simulink model "Fuel_Cell"  (R2023b)
settings: Solver=ode1  StartTime=0.0  StopTime=100  FixedStep=0.02  RelTol=1e-3  AbsTol=1e-3  EnableMultiTasking=on
model workspace: external: MATLAB File model_workspace.m (data not in the file)
values from neighbouring files (symbols this model uses):
  anode_tube_D = 0.004    [model_workspace.m]
  cathode_tube_D = 0.004    [model_workspace.m]
  env_p = 0.101325    [model_workspace.m]
  env_T = 60    [model_workspace.m]
  Ki_valve = 0.0005    [model_workspace.m]
  Kp_valve = 5E-5    (= 5e-05)    [model_workspace.m]
  N2_T = [-56.55 -50 -40 -30 -20 -10 -5 -4 -3 -2 -1 0 1 2 3 4 5 10 20 30          40 50 60 70 80 90 100 110 120 130 140 150 160 170 180 190 200 210          220 230 240 250 260 270 280 290 300 310 320 330 340 350]    [model_workspace.m]
  radiator_air_area_fins = 11.5625    [model_workspace.m]
  radiator_air_area_primary = 1.2231250000000002    (= 1.223125)    [model_workspace.m]
  radiator_eta_fin = 0.7    [model_workspace.m]
  radiator_rho = 2700    [model_workspace.m]
  radiator_t_wall = 0.0001    [model_workspace.m]
  stack_area = 49    [model_workspace.m]
  stack_iL = 1.4    [model_workspace.m]
  stack_mea_rho = 1800    [model_workspace.m]
  stack_num_cells = 8    [model_workspace.m]
  stack_num_channels = 1    [model_workspace.m]
  stack_t_gdl = 250    [model_workspace.m]
  stack_t_membrane = 125    [model_workspace.m]
  stack_w_channels = 0.4    [model_workspace.m]
  time_step = 0.02    [model_workspace.m]
libraries: fl_lib x108, nesl_utility x48, simulink x10
(part 1 of 3)
settings Model: Creator=The MathWorks, Inc.  LastModifiedBy=danie
settings ConfigSet: Description=VeriStand Targets (Windows & NI Linux Real-Time 64-bit)
settings SolverCC: AutoScaleAbsTol=off  MaxConsecutiveMinStep=2  AlgebraicLoopSolver=TrustRegion  AutoInsertRateTranBlk=on  InsertRTBMode=Always  MaxZcPerStep=1
settings DataIOCC: SaveOutput=off  SaveTime=off  ReturnWorkspaceOutputs=off
settings OptimizationCC: DefaultParameterBehavior=Inlined  EnhancedBackFolding=on  PassReuseOutputArgsAs=Individual arguments  ZeroExternalMemoryAtStartup=off  ZeroInternalMemoryAtStartup=off  OptimizeBlockOrder=speed  DifferentSizesBufferReuse=on  OptimizationCustomize=off  EfficientTunableParamExpr=on
settings DebuggingCC: ParameterTunabilityLossMsg=error  UnconnectedInputMsg=warning  UnconnectedOutputMsg=warning  UnconnectedLineMsg=warning  SymbolicDimsDataTypeCodeGenerationDiagnostic=none
settings HardwareCC: ProdBitPerLong=64  ProdHWDeviceType=Intel->x86-64 (Linux 64)
settings ModelReferenceCC: EnableRefExpFcnMdlSchedulingChecks=on
settings SFSimCC: MATLABDynamicMemAlloc=off  CustomCodeUndefinedFunction=UseInterfaceOnly
settings RTWCC: Description=Embedded Coder  SystemTargetFile=ert.tlc  GenCodeOnly=on  PackageGeneratedCodeAndArtifacts=on  TemplateMakefile=ert_default_tmf  BuildConfiguration=Faster Runs  DLArmComputeVersion=19.05
settings CodeAppCC: ForceParamTrailComments=on  IgnoreCustomStorageClasses=off  OperatorAnnotations=on  SimulinkDataObjDesc=on  SFDataObjDesc=on  InsertBlockDesc=on
settings ERTTargetCC: TargetLangStandard=C99 (ISO)  GenerateSampleERTMain=on  SupportContinuousTime=on  InlinedParameterPlacement=NonHierarchical  ERTCustomFileTemplate=example_file_process.tlc
settings SimscapeCC: SimscapeLogName=simlog_ssc_fuel_cell  SimscapeLogDataHistory=20000

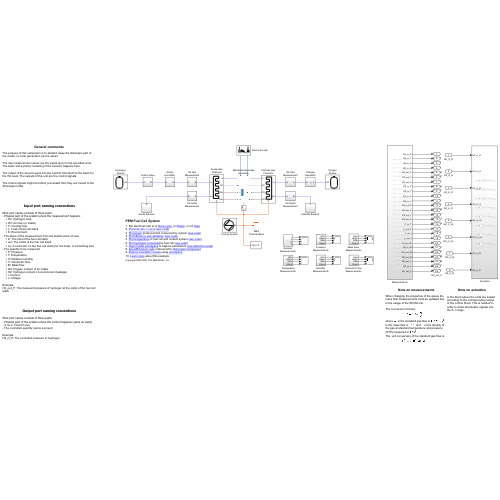
[thumbnail: Simulink's stored preview of the top-level diagram]
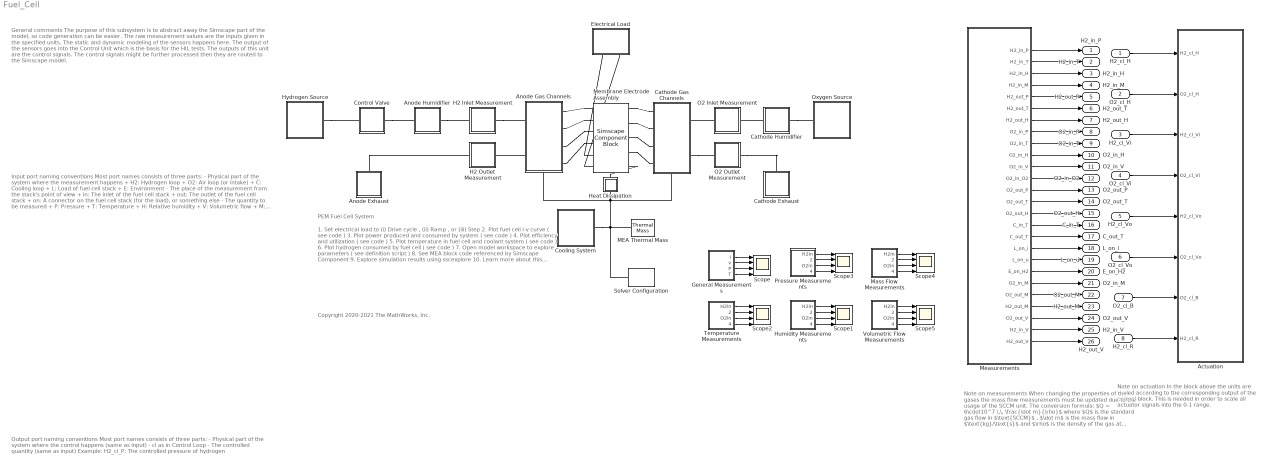
== system Fuel_Cell ==
  note: Note on actuation
      |
      | In the block above the units are scaled according to the corresponding output of the control block. This is needed in order to scale all actuator signals into the 0-1 range.
  note: Note on measurements
      |
      | When changing the properties of the gases the mass flow measurements must be updated due to the usage of the SCCM unit.
      |
      | The conversion formula:
      | $Q = 6\cdot10^7 \,\, \frac{\dot m}{\rho}$
      | where $Q$ is the standard gas flow in $\text{SCCM}$ , $\dot m$ is the mass flow in $\text{kg}/\text{s}$ and $\rho$ is the density of the gas at standard temperature and pressure (STP) measured in ${\text{kg}}/{\text{m}^3}$ .
      | The unit conversion of the standard gas flow is
      | $1 \frac{\text{m}^3}{\text{s}} = 6\cdot10^7 \,\,\text{SCCM}$
  note: PEM Fuel Cell System
  note: 1. Set electrical load to (i) Drive cycle , (ii) Ramp , or (iii) Step
      | 2. Plot fuel cell i-v curve ( see code )
      | 3. Plot power produced and consumed by system ( see code )
      | 4. Plot efficiency and utilization ( see code )
      | 5. Plot temperature in fuel cell and coolant system ( see code )
      | 6. Plot hydrogen consumed by fuel cell ( see code )
      | 7. Open model workspace to explore parameters ( see definition script )
      | 8. See MEA block code referenced by Simscape Component
      | 9. Explore simulation results using sscexplore
      | 10. Learn more about this example
  note: Copyright 2020-2021 The MathWorks, Inc.
  note: General comments
      |
      | The purpose of this subsystem is to abstract away the Simscape part of the model, so code generation can be easier.
      |
      | The raw measurement values are the inputs given in the specified units. The static and dynamic modeling of the sensors happens here.
      |
      | The output of the sensors goes into the Control Unit which is the basis for the HIL tests. The outputs of this unit are the control signals.
      |
      | The control signals might be further processed then they are routed to the Simscape model.
  note: Input port naming conventions
      |
      | Most port names consists of three parts:
      | - Physical part of the system where the measurement happens
      | + H2: Hydrogen loop
      | + O2: Air loop (or intake)
      | + C: Cooling loop
      | + L: Load of fuel cell stack
      | + E: Environment
      | - The place of the measurement from the stack's point of view
      | + in: The inlet of the fuel cell stack
      | + out: The outlet of the fuel cell stack
      | + on: A connector on the fuel cell stack (for the load), or something else
      | - The quantity to be measured
      | + P: Pressure
      | + T: Temperature
      | + H: Relative humidity
      | + V: Volumetric flow
      | + M: Mass flow
      | + O2: Oxygen content of air intake
      | + H2: Hydrogen content of environment (leakage)
      | + i: Current
      | + u: Voltage
      |
      | Example:
      | H2_out_P: The measuerd pressure of hydrogen at the outlet of the fuel cell stack
  note: Output port naming conventions
      |
      | Most port names consists of three parts:
      | - Physical part of the system where the control happens (same as input)
      | - cl as in Control Loop
      | - The controlled quantity (same as input)
      |
      | Example:
      | H2_cl_P: The controlled pressure of hydrogen
  H2_cl_H : Inport  OutDataTypeStr=double  PortDimensions=[1 1]  SampleTime=[time_step,0]
  O2_cl_H : Inport  Port=2  OutDataTypeStr=double  PortDimensions=[1 1]  SampleTime=[time_step,0]
  H2_cl_Vi : Inport  Port=3  OutDataTypeStr=double  PortDimensions=1  SampleTime=[time_step,0]
  O2_cl_Vi : Inport  Port=4  OutDataTypeStr=double  PortDimensions=1  SampleTime=[time_step,0]
  H2_cl_Vo : Inport  Port=5  OutDataTypeStr=double  PortDimensions=1  SampleTime=[time_step,0]
  O2_cl_Vo : Inport  Port=6  OutDataTypeStr=double  PortDimensions=1  SampleTime=[time_step,0]
  O2_cl_B : Inport  Port=7  OutDataTypeStr=double  PortDimensions=1  SampleTime=[time_step,0]
  H2_cl_R : Inport  Port=8  OutDataTypeStr=double  PortDimensions=1  SampleTime=[time_step,0]
  Actuation : Subsystem
  Anode Humidifier : Subsystem  Tag=PublishSubsystem
  Anode Exhaust : Subsystem  Tag=PublishSubsystem
      settings: PortSchema="{\"entries\":[{\"content\":{\"sides\":[{\"content\":{\"connectorIds\":[]},\"type\":\"ConnectorPlacement.EquallySpacedRectSide\",\"uuid\":\"6344d1cf-22ea-4a51-9588-07afca0fac15\"},{\"content\":{\"connectorIds\":[],\"side\":\"RIGHT\"},\"type\":\"ConnectorPlacement.EquallySpacedRectSide\",\"uuid\":\"a3908f81-9410-4056-87cd-9faba76d3fb8\"},{\"content\":{\"connectorIds\":[\"LConn1\"],\"side\":\"TOP\"},\"type\":\"ConnectorPlacement.EquallySpacedRectSide\",\"uuid\":\"a1c9e24d-adb9-4361-8e9b-feafccbbdb81\"}]},\"type\":\"ConnectorPlacement.EquallySpacedConnector\",\"uuid\":\"d5180d8f-18a0-491d-9fff-909db43c9aea\"}],\"packageUris\":[\"http://schema.mathworks.com/mf0/Connector/R2020b\"],\"version\":\"1.0\"}"
  Anode Gas Channels : Subsystem  Tag=PublishSubsystem
      settings: PortSchema="{\"entries\":[{\"content\":{\"sides\":[{\"content\":{\"connectorIds\":[\"LConn1\",\"LConn2\"]},\"type\":\"ConnectorPlacement.EquallySpacedRectSide\",\"uuid\":\"f0c92738-2de1-40ac-9e4a-670524600aa2\"},{\"content\":{\"connectorIds\":[\"RConn1\",\"RConn2\",\"RConn3\",\"RConn4\"],\"side\":\"RIGHT\"},\"type\":\"ConnectorPlacement.EquallySpacedRectSide\",\"uuid\":\"f0ed995d-2dce-4bd6-9faa-b1cb502a30b1\"},{\"content\":{\"connectorIds\":[],\"side\":\"TOP\"},\"type\":\"ConnectorPlacement.EquallySpacedRectSide\",\"uuid\":\"b5d2d698-46b6-42b5-a767-bb9f1790aa28\"},{\"content\":{\"connectorIds\":[\"RConn5\"],\"side\":\"BOTTOM\"},\"type\":\"ConnectorPlacement.EquallySpacedRectSide\",\"uuid\":\"3e8c99a3-0044-43a9-bacb-b652445e4ac6\"}]},\"type\":\"ConnectorPlacement.EquallySpacedConnector\",\"uuid\":\"912925fb-ca80-4fe6-8a1d-a2308cfd6f88\"}],\"packageUris\":[\"http://schema.mathworks.com/mf0/Connector/R2020b\"],\"version\":\"1.0\"}"
      mask Display:
      | plot(0, 0)
      | plot(100, 100)
      | 
      | x1 = 25;
      | x2 = 65;
      | y1 = 23;
      | y2 = 95;
      | xt = 15;
      | yt = 9;
      | 
      | x_pattern = [x2 x2    x1+xt x1+xt   x1+xt   x2     ];
      | y_pattern = [y2 y2-yt y2-yt y2-2*yt y2-2*yt y2-2*yt];
      | 
      | plot([x1 x1 x2 x_pattern x_pattern      x_pattern      x_pattern         x2    x1], ...
      |      [y1-yt y2 y2 y_pattern y_pattern-2*yt y_pattern-4*yt y_pattern-6*yt y1-yt y1-yt])
  Cathode Humidifier : Subsystem  Tag=PublishSubsystem
  Cathode Exhaust : Subsystem  Tag=PublishSubsystem
      settings: PortSchema="{\"entries\":[{\"content\":{\"sides\":[{\"content\":{\"connectorIds\":[]},\"type\":\"ConnectorPlacement.EquallySpacedRectSide\",\"uuid\":\"6344d1cf-22ea-4a51-9588-07afca0fac15\"},{\"content\":{\"connectorIds\":[],\"side\":\"RIGHT\"},\"type\":\"ConnectorPlacement.EquallySpacedRectSide\",\"uuid\":\"a3908f81-9410-4056-87cd-9faba76d3fb8\"},{\"content\":{\"connectorIds\":[\"LConn1\"],\"side\":\"TOP\"},\"type\":\"ConnectorPlacement.EquallySpacedRectSide\",\"uuid\":\"a1c9e24d-adb9-4361-8e9b-feafccbbdb81\"}]},\"type\":\"ConnectorPlacement.EquallySpacedConnector\",\"uuid\":\"d5180d8f-18a0-491d-9fff-909db43c9aea\"}],\"packageUris\":[\"http://schema.mathworks.com/mf0/Connector/R2020b\"],\"version\":\"1.0\"}"
  Cathode Gas Channels : Subsystem  Tag=PublishSubsystem
      settings: PortSchema="{\"entries\":[{\"content\":{\"sides\":[{\"content\":{\"connectorIds\":[\"LConn1\",\"LConn2\",\"LConn3\",\"LConn4\"]},\"type\":\"ConnectorPlacement.EquallySpacedRectSide\",\"uuid\":\"d09155df-6760-40de-80f3-d532399b6b43\"},{\"content\":{\"connectorIds\":[\"RConn1\",\"RConn2\"],\"side\":\"RIGHT\"},\"type\":\"ConnectorPlacement.EquallySpacedRectSide\",\"uuid\":\"8f76bd4e-30c2-4c8b-860a-78c10353bd22\"},{\"content\":{\"connectorIds\":[],\"side\":\"TOP\"},\"type\":\"ConnectorPlacement.EquallySpacedRectSide\",\"uuid\":\"7de91a32-4f26-479e-bbec-b6009a288b8f\"},{\"content\":{\"connectorIds\":[\"RConn3\"],\"side\":\"BOTTOM\"},\"type\":\"ConnectorPlacement.EquallySpacedRectSide\",\"uuid\":\"b696b46e-4734-4c8a-bae1-7c8793078c6b\"}]},\"type\":\"ConnectorPlacement.EquallySpacedConnector\",\"uuid\":\"30d7c265-b676-4649-8112-8a94c6c095da\"}],\"packageUris\":[\"http://schema.mathworks.com/mf0/Connector/R2020b\"],\"version\":\"1.0\"}"
      mask Display:
      | plot(0, 0)
      | plot(100, 100)
      | 
      | x1 = 35;
      | x2 = 75;
      | y1 = 23;
      | y2 = 95;
      | xt = 15;
      | yt = 9;
      | 
      | x_pattern = [x1 x1    x2-xt x2-xt   x2-xt   x1     ];
      | y_pattern = [y2 y2-yt y2-yt y2-2*yt y2-2*yt y2-2*yt];
      | 
      | plot([x2 x2 x1 x_pattern x_pattern      x_pattern      x_pattern         x1    x2], ...
      |      [y1-yt y2 y2 y_pattern y_pattern-2*yt y_pattern-4*yt y_pattern-6*yt y1-yt y1-yt])
  Control Valve : Subsystem  Tag=PublishSubsystem
  Cooling System : Subsystem  Tag=PublishSubsystem
      mask Display:
      | plot(0, 0)
      | plot(100, 100)
      | 
      | n = 80;
      | r = 35;
      | 
      | x = 45;
      | y = 50;
      | t = 5;
      | 
      | plot(cos(linspace(0, 2*pi, n))*r + x, sin(linspace(0, 2*pi, n))*r + y)
      | 
      | plot([x x x-r+t x+r-t x x], [y+r+2*t y+r-t y y y-r+t y-r-2*t])
  Electrical Load : Subsystem  Tag=PublishSubsystem  mask(Electrical Load){input_type=Drive cycle}
      mask prompts: input_type "Select one of the following scenarios:"
      settings: PortSchema="{\"entries\":[{\"content\":{\"sides\":[{\"content\":{\"connectorIds\":[]},\"type\":\"ConnectorPlacement.EquallySpacedRectSide\",\"uuid\":\"cf26c57a-4aaa-4eca-a1cf-dab3379228b7\"},{\"content\":{\"connectorIds\":[],\"side\":\"RIGHT\"},\"type\":\"ConnectorPlacement.EquallySpacedRectSide\",\"uuid\":\"bd4a28c6-f8d3-4492-9f61-a12eb17ccdd3\"},{\"content\":{\"connectorIds\":[],\"side\":\"TOP\"},\"type\":\"ConnectorPlacement.EquallySpacedRectSide\",\"uuid\":\"7f54a4db-ccf4-4e3a-a135-4ada067d241f\"},{\"content\":{\"connectorIds\":[\"RConn1\",\"RConn2\"],\"side\":\"BOTTOM\"},\"type\":\"ConnectorPlacement.EquallySpacedRectSide\",\"uuid\":\"8817983d-3f79-43b3-9594-6d12f7dcf066\"}]},\"type\":\"ConnectorPlacement.EquallySpacedConnector\",\"uuid\":\"79253ea6-cd7f-4983-840a-f5cee3a4dd91\"}],\"packageUris\":[\"http://schema.mathworks.com/mf0/Connector/R2020b\"],\"version\":\"1.0\"}"
      mask TypeOptions input_type: Drive cycle | Current Ramp | Current Step | Current Ramped Step | Power Ramped Step
      mask Callback input_type:
      | activeVariant = get_param(gcb, 'input_type');
      | set_param([gcb '/Inputs'], 'OverrideUsingVariant', activeVariant)
      mask Display:
      | blk = get_param([gcb, '/Inputs'], 'CompiledActiveChoiceBlock');
      | eval(get_param(blk, 'MaskDisplay'))
  General Measurements : Subsystem
  H2 Inlet Measurement : Subsystem  Tag=PublishSubsystem
  H2 Outlet Measurement : Subsystem  Tag=PublishSubsystem
  Heat Dissipation : Subsystem
      settings: PortSchema="{\"entries\":[{\"content\":{\"sides\":[{\"content\":{\"connectorIds\":[]},\"type\":\"ConnectorPlacement.EquallySpacedRectSide\",\"uuid\":\"40b2385a-b20e-464f-8016-3228e4acac4a\"},{\"content\":{\"connectorIds\":[],\"side\":\"RIGHT\"},\"type\":\"ConnectorPlacement.EquallySpacedRectSide\",\"uuid\":\"0e95dc4b-d2da-4ab6-a6e9-e2cb275776ce\"},{\"content\":{\"connectorIds\":[\"LConn1\"],\"side\":\"TOP\"},\"type\":\"ConnectorPlacement.EquallySpacedRectSide\",\"uuid\":\"0f5995c7-26f6-433d-889b-dea78bcd2b2a\"},{\"content\":{\"connectorIds\":[\"RConn1\"],\"side\":\"BOTTOM\"},\"type\":\"ConnectorPlacement.EquallySpacedRectSide\",\"uuid\":\"a2ee1c19-f9e9-4dbd-a9ff-92feea387e85\"}]},\"type\":\"ConnectorPlacement.EquallySpacedConnector\",\"uuid\":\"721753ea-9ada-4c74-8c6f-50b905d96904\"}],\"packageUris\":[\"http://schema.mathworks.com/mf0/Connector/R2020b\"],\"version\":\"1.0\"}"
  Humidity Measurements : Subsystem
  Hydrogen Source : Subsystem  Tag=PublishSubsystem
      mask Display:
      | plot(0, 0)
      | plot(100, 100)
      | 
      | n = 20;
      | r = 20;
      | x1 = 15;
      | x2 = 65;
      | y1 = 5;
      | y2 = 85;
      | 
      | plot([x1 x1], [y1+r y2-r])
      | plot([x1+r x2-r], [y2 y2])
      | plot([x2 x2], [y2-r y1+r])
      | plot([x2-r x1+r], [y1 y1])
      | 
      | plot(cos(linspace(pi/2, pi, n))*r + x1+r, sin(linspace(pi/2, pi, n))*r + y2-r)
      | plot(cos(linspace(0, pi/2, n))*r + x2-r, sin(linspace(0, pi/2, n))*r + y2-r)
      | plot(cos(linspace(3*pi/2, 2*pi, n))*r + x2-r, sin(linspace(3*pi/2, 2*pi, n))*r + y1+r)
      | plot(cos(linspace(pi, 3*pi/2, n))*r + x1+r, sin(linspace(pi, 3*pi/2, n))*r + y1+r)
      | 
      | plot([-5 -5 5 5] + (x1+x2)/2, [0 5 5 0] + y2)
  MEA Thermal Mass : fl_lib/Thermal/Thermal Elements/Thermal Mass  mass_type=foundation.enum.constant_variable.constant  mass=stack_mea_rho * stack_area*1e-4 * (stack_t_membrane + 2*stack_t_gdl)*1e-6 * stack_num_cells kg  sp_heat=stack_mea_cp J/kg/K  mass_min=1e-6 kg  num_ports=foundation.enum.numPorts2.one  m_specify=off  m_priority=High  m=1 kg  m_nominal_specify=off  m_nominal_unit=kg  m_nominal_value=1  T_specify=on  T_priority=High  T=env_T degC  T_nominal_specify=off  T_nominal_unit=K  T_nominal_value=1  Q_specify=off  Q_priority=None  Q=0 W  Q_nominal_specify=off  Q_nominal_unit=W  Q_nominal_value=1
  Mass Flow Measurements : Subsystem
  Measurements : Subsystem
  Membrane Electrode Assembly : SimscapeComponentBlock  SourceFile=FuelCell  ComponentPath=FuelCell  ComponentVariants="[\"FuelCell\"]"  ComponentVariantNames="[\"FuelCell\"]"  ClassName=FuelCell  SchemaVersion=1  N_cell=stack_num_cells  area_cell=stack_area cm^2  t_membrane=stack_t_membrane um  t_gdl_A=stack_t_gdl um  t_gdl_C=stack_t_gdl um  io=stack_io A/cm^2  iL=stack_iL A/cm^2  alpha=stack_alpha  D_H2O_gdl_A=stack_D_gdl cm^2/s  D_H2O_gdl_C=stack_D_gdl cm^2/s  rho_membrane=stack_membrane_rho kg/m^3  M_membrane=stack_membrane_MW kg/mol  i_specify=off  i_priority=None  i=0 A  i_nominal_specify=off  i_nominal_unit=A  i_nominal_value=1  Q_specify=off  Q_priority=None  Q=0 W  Q_nominal_specify=off  Q_nominal_unit=W  Q_nominal_value=1  a_H2O_acl_specify=off  a_H2O_acl_priority=None  a_H2O_acl=0.5  a_H2O_acl_nominal_specify=off  a_H2O_acl_nominal_unit=1  a_H2O_acl_nominal_value=1  a_H2O_ccl_specify=off  a_H2O_ccl_priority=None  a_H2O_ccl=0.5  a_H2O_ccl_nominal_specify=off  a_H2O_ccl_nominal_unit=1  a_H2O_ccl_nominal_value=1
      settings: CopyFcn=simscape.engine.sli.internal.componentblockcallback(gcbh,'COPY')  PreCopyFcn=simscape.engine.sli.internal.componentblockcallback(gcbh,'PRECOPY')  PreDeleteFcn=simscape.engine.sli.internal.componentblockcallback(gcbh,'PREDELETE')  InternalSimscapePortConfiguration="{\"Bottom\":[{\"id\":\"H\",\"label\":\"H\",\"type\":\"foundation.thermal.thermal\"}],\"Left\":[{\"id\":\"A\",\"label\":\"A\",\"type\":\"foundation.moist_air.moist_air\"},{\"id\":\"SA\",\"label\":\"SA\",\"type\":\"foundation.moist_air.moist_air_source\"},{\"id\":\"FAi\",\"label\":\"FAi\",\"type\":\"input\"},{\"id\":\"FAo\",\"label\":\"FAo\",\"type\":\"input\"}],\"Right\":[{\"id\":\"C\",\"label\":\"C\",\"type\":\"foundation.moist_air.moist_air\"},{\"id\":\"SC\",\"label\":\"SC\",\"type\":\"foundation.moist_air.moist_air_source\"},{\"id\":\"FCi\",\"label\":\"FCi\",\"type\":\"input\"},{\"id\":\"FCo\",\"label\":\"FCo\",\"type\":\"input\"}],\"Top\":[{\"id\":\"n\",\"label\":\"-\",\"type\":\"foundation.electrical.electrical\"},{\"id\":\"p\",\"label\":\"+\",\"type\":\"foundation.electrical.electrical\"}]}"
      mask Type: Fuel Cell
  O2 Inlet Measurement : Subsystem  Tag=PublishSubsystem
  O2 Outlet Measurement : Subsystem  Tag=PublishSubsystem
  Oxygen Source : Subsystem  Tag=PublishSubsystem
      mask Display:
      | plot(0, 0)
      | plot(100, 100)
      | 
      | n = 20;
      | r = 20;
      | x1 = 35;
      | x2 = 85;
      | y1 = 5;
      | y2 = 85;
      | 
      | plot([x1 x1], [y1+r y2-r])
      | plot([x1+r x2-r], [y2 y2])
      | plot([x2 x2], [y2-r y1+r])
      | plot([x2-r x1+r], [y1 y1])
      | 
      | plot(cos(linspace(pi/2, pi, n))*r + x1+r, sin(linspace(pi/2, pi, n))*r + y2-r)
      | plot(cos(linspace(0, pi/2, n))*r + x2-r, sin(linspace(0, pi/2, n))*r + y2-r)
      | plot(cos(linspace(3*pi/2, 2*pi, n))*r + x2-r, sin(linspace(3*pi/2, 2*pi, n))*r + y1+r)
      | plot(cos(linspace(pi, 3*pi/2, n))*r + x1+r, sin(linspace(pi, 3*pi/2, n))*r + y1+r)
      | 
      | plot([-5 -5 5 5] + (x1+x2)/2, [0 5 5 0] + y2)
  Pressure Measurements : Subsystem
  Scope{,1..5} (6 alike) : Scope  NumInputPorts=4
  Solver Configuration : nesl_utility/Solver Configuration  PhysicalDomain=network_engine_domain  SubClassName=solver  LeftPortType=input  RightPortType=generic  Tones=[]  Harmonics=[]  SimulateNoise=off  Profile=off  UseLocalSampling=off  EnableSwitchedLinearOptims=on  FrequencyDomain=off  UseCCode=off  RelTol=0.001  AbsTol=1e-06  MinStep=1e-09  ToWorkspace=off  RevertToSquareIcSolve=off  NumHomotopyIterations=100  PhasorMode=off  PhasorModeNumHarmonics=1  ConsistencySolver=NEWTON_FTOL  IndexReductionMethod=DerivativeReplacement  DoDC=on  ResidualTolerance=1e-05  ConsistencyTolSource=GLOBAL  ConsistencyAbsTol=0.001  ConsistencyRelTol=0.001  ConsistencyTolFactor=0.001  UseLocalSolver=on  LocalSolverChoice=NE_BACKWARD_EULER_ADVANCER  ResolveIndetEquations=on  FunctionEvalNumThread=1  LocalSolverSampleTime=time_step  DoFixedCost=off  MaxNonlinIter=3  MaxModeIter=2  ComputeImpulses=off  ImpulseIterations=2  LinearAlgebra=auto  LinearAlgebraNumThread=0  EquationFormulation=NE_TIME_EF  DelaysMemoryBudget=1024  AutomaticFiltering=on  FilteringTimeConstant=0.01  PartitionStorageMethod=AS_NEEDED  PartitionMemoryBudget=1024  PartitionMethod=ROBUST  MultibodyUseLocalSolver=off  MultibodyLocalSolverChoice=ODE1  MultibodyLocalSolverSampleTime=0.001
  Temperature Measurements : Subsystem
  Volumetric Flow Measurements : Subsystem
  H2_in_P : Outport  OutDataTypeStr=double  PortDimensions=[1 1]  SampleTime=[time_step,0]
  H2_in_T : Outport  Port=2  OutDataTypeStr=double  PortDimensions=[1 1]  SampleTime=[time_step,0]
  H2_in_H : Outport  Port=3  OutDataTypeStr=double  PortDimensions=[1 1]  SampleTime=[time_step,0]
  H2_in_M : Outport  Port=4  OutDataTypeStr=double  PortDimensions=[1 1]  SampleTime=[time_step,0]
  H2_out_P : Outport  Port=5  OutDataTypeStr=double  PortDimensions=[1 1]  SampleTime=[time_step,0]
  H2_out_T : Outport  Port=6  OutDataTypeStr=double  PortDimensions=[1 1]  SampleTime=[time_step,0]
  H2_out_H : Outport  Port=7  OutDataTypeStr=double  PortDimensions=[1 1]  SampleTime=[time_step,0]
  O2_in_P : Outport  Port=8  OutDataTypeStr=double  PortDimensions=[1 1]  SampleTime=[time_step,0]
  O2_in_T : Outport  Port=9  OutDataTypeStr=double  PortDimensions=[1 1]  SampleTime=[time_step,0]
  O2_in_H : Outport  Port=10  OutDataTypeStr=double  PortDimensions=[1 1]  SampleTime=[time_step,0]
  O2_in_V : Outport  Port=11  OutDataTypeStr=double  PortDimensions=[1 1]  SampleTime=[time_step,0]
  O2_in_O2 : Outport  Port=12  OutDataTypeStr=double  PortDimensions=[1 1]  SampleTime=[time_step,0]
  O2_out_P : Outport  Port=13  OutDataTypeStr=double  PortDimensions=[1 1]  SampleTime=[time_step,0]
  O2_out_T : Outport  Port=14  OutDataTypeStr=double  PortDimensions=[1 1]  SampleTime=[time_step,0]
  O2_out_H : Outport  Port=15  OutDataTypeStr=double  PortDimensions=[1 1]  SampleTime=[time_step,0]
  C_in_T : Outport  Port=16  OutDataTypeStr=double  PortDimensions=1  SampleTime=[time_step,0]
  C_out_T : Outport  Port=17  OutDataTypeStr=double  PortDimensions=1  SampleTime=[time_step,0]
  L_on_i : Outport  Port=18  OutDataTypeStr=double  PortDimensions=1  SampleTime=[time_step,0]
  L_on_u : Outport  Port=19  OutDataTypeStr=double  PortDimensions=1  SampleTime=[time_step,0]
  E_on_H2 : Outport  Port=20  OutDataTypeStr=double  PortDimensions=1  SampleTime=[time_step,0]
  O2_in_M : Outport  Port=21  OutDataTypeStr=double  PortDimensions=[1 1]  SampleTime=[time_step,0]
  O2_out_M : Outport  Port=22  OutDataTypeStr=double  PortDimensions=[1 1]  SampleTime=[time_step,0]
  H2_out_M : Outport  Port=23  OutDataTypeStr=double  PortDimensions=[1 1]  SampleTime=[time_step,0]
  O2_out_V : Outport  Port=24  OutDataTypeStr=double  PortDimensions=[1 1]  SampleTime=[time_step,0]
  H2_in_V : Outport  Port=25  OutDataTypeStr=double  PortDimensions=[1 1]  SampleTime=[time_step,0]
  H2_out_V : Outport  Port=26  OutDataTypeStr=double  PortDimensions=[1 1]  SampleTime=[time_step,0]
  wires:
  H2_cl_Vi/1 -> Actuation/3(H2_cl_Vi)
  Temperature Measurements/2(H2out) -> Scope2/2
  Pressure Measurements/1(H2in) -> Scope3/1
  General Measurements/3(P) -> Scope/3
  Measurements/7(H2_out_H) -> H2_out_H/1
  Measurements/14(O2_out_T) -> O2_out_T/1
  Temperature Measurements/3(O2in) -> Scope2/3
  Measurements/13(O2_out_P) -> O2_out_P/1
  Measurements/21(O2_in_M) -> O2_in_M/1
  Pressure Measurements/4(O2out) -> Scope3/4
  General Measurements/2(v) -> Scope/2
  Humidity Measurements/2(H2out) -> Scope1/2
  General Measurements/4(T) -> Scope/4
  Measurements/26(H2_out_V) -> H2_out_V/1
  Volumetric Flow Measurements/4(O2out) -> Scope5/4
  Measurements/10(O2_in_H) -> O2_in_H/1
  Pressure Measurements/2(H2out) -> Scope3/2
  Humidity Measurements/1(H2in) -> Scope1/1
  Volumetric Flow Measurements/1(H2in) -> Scope5/1
  O2_cl_H/1 -> Actuation/2(O2_cl_H)
  Measurements/22(O2_out_M) -> O2_out_M/1
  Mass Flow Measurements/3(O2in) -> Scope4/3
  Measurements/12(O2_in_O2) -> O2_in_O2/1
  Volumetric Flow Measurements/2(H2out) -> Scope5/2
  Measurements/3(H2_in_H) -> H2_in_H/1
  Mass Flow Measurements/2(H2out) -> Scope4/2
  Pressure Measurements/3(O2in) -> Scope3/3
  Humidity Measurements/4(O2out) -> Scope1/4
  Mass Flow Measurements/1(H2in) -> Scope4/1
  Measurements/9(O2_in_T) -> O2_in_T/1
  H2_cl_H/1 -> Actuation/1(H2_cl_H)
  Mass Flow Measurements/4(O2out) -> Scope4/4
  Volumetric Flow Measurements/3(O2in) -> Scope5/3
  Temperature Measurements/4(O2out) -> Scope2/4
  Humidity Measurements/3(O2in) -> Scope1/3
  General Measurements/1(i) -> Scope/1
  Temperature Measurements/1(H2in) -> Scope2/1
  Measurements/4(H2_in_M) -> H2_in_M/1
  Measurements/6(H2_out_T) -> H2_out_T/1
  Measurements/2(H2_in_T) -> H2_in_T/1
  Measurements/1(H2_in_P) -> H2_in_P/1
  Measurements/16(C_in_T) -> C_in_T/1
  Measurements/17(C_out_T) -> C_out_T/1
  Measurements/20(E_on_H2) -> E_on_H2/1
  Measurements/11(O2_in_V) -> O2_in_V/1
  Measurements/8(O2_in_P) -> O2_in_P/1
  Measurements/18(L_on_i) -> L_on_i/1
  Measurements/5(H2_out_P) -> H2_out_P/1
  Measurements/15(O2_out_H) -> O2_out_H/1
  Measurements/25(H2_in_V) -> H2_in_V/1
  Measurements/23(H2_out_M) -> H2_out_M/1
  Measurements/19(L_on_u) -> L_on_u/1
  Measurements/24(O2_out_V) -> O2_out_V/1
  O2_cl_Vi/1 -> Actuation/4(O2_cl_Vi)
  H2_cl_Vo/1 -> Actuation/5(H2_cl_Vo)
  O2_cl_Vo/1 -> Actuation/6(O2_cl_Vo)
  O2_cl_B/1 -> Actuation/7(O2_cl_B)
  H2_cl_R/1 -> Actuation/8(H2_cl_R)
  connections:
  MEA Thermal Mass/LConn1 -- Cooling System/RConn1 -- Cathode Gas Channels/RConn3 -- Anode Gas Channels/RConn5 -- Heat Dissipation/RConn1 -- Solver Configuration/RConn1
  Membrane Electrode Assembly/LConn6 -- Electrical Load/RConn2
  Hydrogen Source/RConn1 -- Control Valve/LConn1
  Membrane Electrode Assembly/RConn1 -- Cathode Gas Channels/LConn1
  Membrane Electrode Assembly/LConn2 -- Anode Gas Channels/RConn2
  Anode Exhaust/LConn1 -- H2 Outlet Measurement/LConn1
  Membrane Electrode Assembly/LConn3 -- Anode Gas Channels/RConn3
  Membrane Electrode Assembly/RConn2 -- Cathode Gas Channels/LConn2
  Membrane Electrode Assembly/LConn4 -- Anode Gas Channels/RConn4
  Cathode Gas Channels/RConn2 -- O2 Outlet Measurement/LConn1
  Cathode Humidifier/RConn1 -- Oxygen Source/RConn1
  Membrane Electrode Assembly/RConn5 -- Heat Dissipation/LConn1
  O2 Outlet Measurement/RConn1 -- Cathode Exhaust/LConn1
  Membrane Electrode Assembly/LConn1 -- Anode Gas Channels/RConn1
  H2 Inlet Measurement/RConn1 -- Anode Gas Channels/LConn1
  O2 Inlet Measurement/LConn1 -- Cathode Gas Channels/RConn1
  Cathode Humidifier/LConn1 -- O2 Inlet Measurement/RConn1
  Anode Gas Channels/LConn2 -- H2 Outlet Measurement/RConn1
  Membrane Electrode Assembly/RConn3 -- Cathode Gas Channels/LConn3
  Membrane Electrode Assembly/LConn5 -- Electrical Load/RConn1
  Membrane Electrode Assembly/RConn4 -- Cathode Gas Channels/LConn4
  Anode Humidifier/RConn1 -- H2 Inlet Measurement/LConn1
  Control Valve/RConn1 -- Anode Humidifier/LConn1

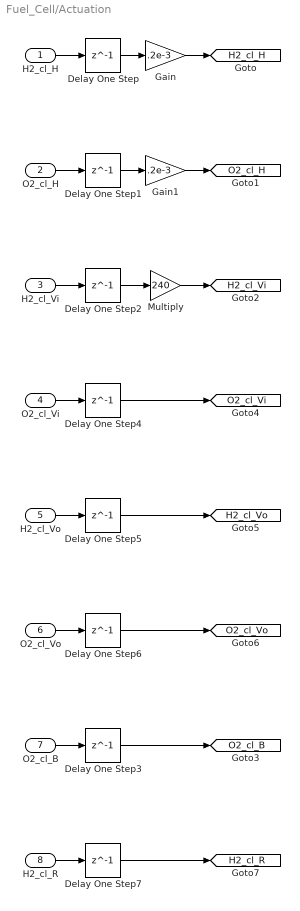
== system Fuel_Cell/Actuation ==
  H2_cl_H : Inport
  O2_cl_H : Inport  Port=2
  H2_cl_Vi : Inport  Port=3
  O2_cl_Vi : Inport  Port=4
  H2_cl_Vo : Inport  Port=5
  O2_cl_Vo : Inport  Port=6
  O2_cl_B : Inport  Port=7
  H2_cl_R : Inport  Port=8
  Delay One Step{,1..7} (8 alike) : Delay  DelayLength=1
  Gain : Gain  Gain=.2e-3
  Gain1 : Gain  Gain=.2e-3
  Multiply : Gain  Gain=240
  tag scope: H2_cl_H=global, H2_cl_R=global, H2_cl_Vi=global, H2_cl_Vo=global, O2_cl_B=global, O2_cl_H=global, O2_cl_Vi=global, O2_cl_Vo=global
  wires:
  Delay One Step4/1 -> [O2_cl_Vi]
  Delay One Step3/1 -> [O2_cl_B]
  Delay One Step2/1 -> Multiply/1
  Delay One Step1/1 -> Gain1/1
  Delay One Step/1 -> Gain/1
  O2_cl_H/1 -> Delay One Step1/1
  H2_cl_H/1 -> Delay One Step/1
  Gain/1 -> [H2_cl_H]
  Gain1/1 -> [O2_cl_H]
  O2_cl_B/1 -> Delay One Step3/1
  O2_cl_Vi/1 -> Delay One Step4/1
  H2_cl_Vi/1 -> Delay One Step2/1
  Multiply/1 -> [H2_cl_Vi]
  H2_cl_Vo/1 -> Delay One Step5/1
  Delay One Step6/1 -> [O2_cl_Vo]
  O2_cl_Vo/1 -> Delay One Step6/1
  Delay One Step5/1 -> [H2_cl_Vo]
  H2_cl_R/1 -> Delay One Step7/1
  Delay One Step7/1 -> [H2_cl_R]

== system Fuel_Cell/Anode Humidifier ==
  Constant Volume Chamber (MA) : fl_lib/Moist Air/Elements/Constant Volume Chamber (MA)  volume=1 l  num_ports=foundation.enum.num_ports.two  area_A=pi*anode_tube_D^2/4 m^2  area_B=pi*anode_tube_D^2/4 m^2  area_C=0.01 m^2  area_D=0.01 m^2  RH_ws=1  time_constant=1e-3 s  moisture_trace_gas_source=foundation.enum.moisture_trace_gas_source.controlled  moisture_source_spec=foundation.enum.moisture_source_spec.vapor  moisture_mass_flow=0 kg/s  moisture_temperature_spec=foundation.enum.temperature_spec.atmospheric  moisture_temperature=293.15 K  trace_gas_mass_flow=0 kg/s  trace_gas_temperature_spec=foundation.enum.temperature_spec.atmospheric  trace_gas_temperature=293.15 K  p_I_specify=on  p_I_priority=High  p_I=0.101325 MPa  p_I_nominal_specify=off  p_I_nominal_unit=MPa  p_I_nominal_value=1  T_I_specify=on  T_I_priority=High  T_I=env_T degC  T_I_nominal_specify=off  T_I_nominal_unit=K  T_I_nominal_value=1  RH_I_specify=off  RH_I_priority=High  RH_I=0  RH_I_nominal_specify=off  RH_I_nominal_unit=1  RH_I_nominal_value=1  x_w_I_specify=off  x_w_I_priority=None  x_w_I=0  x_w_I_nominal_specify=off  x_w_I_nominal_unit=1  x_w_I_nominal_value=1  y_w_I_specify=off  y_w_I_priority=None  y_w_I=0  y_w_I_nominal_specify=off  y_w_I_nominal_unit=1  y_w_I_nominal_value=1  HR_I_specify=off  HR_I_priority=None  HR_I=0  HR_I_nominal_specify=off  HR_I_nominal_unit=1  HR_I_nominal_value=1  x_g_I_specify=on  x_g_I_priority=None  x_g_I=0  x_g_I_nominal_specify=off  x_g_I_nominal_unit=1  x_g_I_nominal_value=1  y_g_I_specify=on  y_g_I_priority=High  y_g_I=tank_yH2  y_g_I_nominal_specify=off  y_g_I_nominal_unit=1  y_g_I_nominal_value=1
      settings: InternalSimscapePortConfiguration="{\"Bottom\":[],\"Left\":[{\"id\":\"A\",\"label\":\"A\",\"type\":\"foundation.moist_air.moist_air\"},{\"id\":\"B\",\"label\":\"B\",\"type\":\"foundation.moist_air.moist_air\"}],\"Right\":[{\"id\":\"W\",\"label\":\"W\",\"type\":\"output\"},{\"id\":\"F\",\"label\":\"F\",\"type\":\"output\"},{\"id\":\"H\",\"label\":\"H\",\"type\":\"foundation.thermal.thermal\"},{\"id\":\"S\",\"label\":\"S\",\"type\":\"foundation.moist_air.moist_air_source\"}],\"Top\":[]}"
  Controlled Moisture Source (MA) : fl_lib/Moist Air/Sources/Moisture & Trace Gas Sources/Moisture Source (MA)  source_type=foundation.enum.constant_controlled.controlled  moisture_source_spec=foundation.enum.moisture_source_spec.vapor  moisture_mass_flow=0 kg/s  temperature_spec=foundation.enum.temperature_spec.atmospheric  moisture_temperature=293.15 K  Phi_S_specify=off  Phi_S_priority=None  Phi_S=0 kW  Phi_S_nominal_specify=off  Phi_S_nominal_unit=kW  Phi_S_nominal_value=1  mdot_w_S_specify=off  mdot_w_S_priority=None  mdot_w_S=0 kg/s  mdot_w_S_nominal_specify=off  mdot_w_S_nominal_unit=kg/s  mdot_w_S_nominal_value=1
      settings: InternalSimscapePortConfiguration="{\"Bottom\":[],\"Left\":[{\"id\":\"S\",\"label\":\"S\",\"type\":\"foundation.moist_air.moist_air_source\"}],\"Right\":[{\"id\":\"M\",\"label\":\"M\",\"type\":\"input\"},{\"id\":\"T\",\"label\":\"T\",\"type\":\"input\"}],\"Top\":[]}"
  Convective Heat Transfer : fl_lib/Thermal/Thermal Elements/Convective Heat Transfer  thermal_type=foundation.enum.constant_variable.constant  area=0.5 m^2  heat_tr_coeff=900 W/(m^2 * K)  min_heat_tr_coeff=1e-3 W/(K*m^2)  T_specify=off  T_priority=None  T=0 K  T_nominal_specify=off  T_nominal_unit=K  T_nominal_value=1  Q_specify=off  Q_priority=None  Q=0 W  Q_nominal_specify=off  Q_nominal_unit=W  Q_nominal_value=1
  Delay One Step : Delay  DelayLength=1
  Environment Temperature : fl_lib/Thermal/Thermal Sources/Temperature Source  temperature=env_T degC
  Simulink-PS Converter : nesl_utility/Simulink-PS Converter  PhysicalDomain=network_engine_domain  SubClassName=ps_input  LeftPortType=input  RightPortType=output  PseudoPeriodic=off  Frequencies=[]  NoiseDistribution=none  NoiseParameters=[]  Unit=kg/s  AffineConversion=off  FilteringAndDerivatives=provide  SimscapeFilterOrder=1  InputFilterTimeConstant=0.001  UdotUserProvided=0
  Simulink-PS Converter1 : nesl_utility/Simulink-PS Converter  PhysicalDomain=network_engine_domain  SubClassName=ps_input  LeftPortType=input  RightPortType=output  PseudoPeriodic=off  Frequencies=[]  NoiseDistribution=none  NoiseParameters=[]  Unit=degC  AffineConversion=on  FilteringAndDerivatives=provide  SimscapeFilterOrder=1  InputFilterTimeConstant=0.001  UdotUserProvided=0
  A : PMIOPort  Side=Left
  B : PMIOPort  Port=2  Side=Right
  wires:
  Delay One Step/1 -> Simulink-PS Converter1/1
  [H2_cl_H] -> Simulink-PS Converter/1
  [T_stack] -> Delay One Step/1
  connections:
  Environment Temperature/LConn1 -- Convective Heat Transfer/RConn1
  Constant Volume Chamber (MA)/LConn1 -- A/RConn1
  Constant Volume Chamber (MA)/LConn2 -- B/RConn1
  Convective Heat Transfer/LConn1 -- Constant Volume Chamber (MA)/RConn3
  Constant Volume Chamber (MA)/RConn4 -- Controlled Moisture Source (MA)/LConn1
  Simulink-PS Converter1/RConn1 -- Controlled Moisture Source (MA)/RConn2
  Controlled Moisture Source (MA)/RConn1 -- Simulink-PS Converter/RConn1

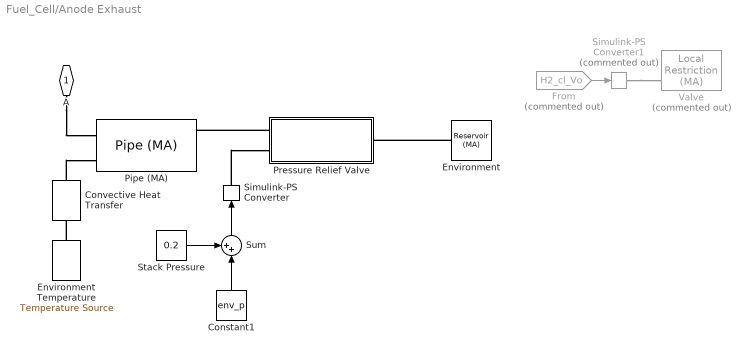
== system Fuel_Cell/Anode Exhaust ==
  Constant1 : Constant  Value=env_p
  Convective Heat Transfer : fl_lib/Thermal/Thermal Elements/Convective Heat Transfer  thermal_type=foundation.enum.constant_variable.constant  area=pi*anode_tube_D*1 m^2  heat_tr_coeff=20 W/(m^2 * K)  min_heat_tr_coeff=1e-3 W/(K*m^2)  T_specify=off  T_priority=None  T=0 K  T_nominal_specify=off  T_nominal_unit=K  T_nominal_value=1  Q_specify=off  Q_priority=None  Q=0 W  Q_nominal_specify=off  Q_nominal_unit=W  Q_nominal_value=1
  Environment : fl_lib/Moist Air/Elements/Reservoir (MA)  pressure_spec=foundation.enum.pressure_spec.specified  reservoir_pressure=env_p MPa  temperature_spec=foundation.enum.temperature_spec.specified  reservoir_temperature=env_T degC  moisture_spec=foundation.enum.moisture_spec.relative_humidity  reservoir_RH=env_RH  reservoir_x_w=0.01  reservoir_y_w=0.01  reservoir_HR=0.01  reservoir_Tw=287 K  trace_gas_spec=foundation.enum.trace_gas_spec.mole_fraction  reservoir_x_g=0.001  reservoir_y_g=env_yO2  RH_ws=1  area_A=pi*cathode_tube_D^2/4 m^2
  Environment Temperature : fl_lib/Thermal/Thermal Sources/Temperature Source  temperature=env_T degC
  From : From  Commented=on  GotoTag=H2_cl_Vo  TagVisibility=global
  Pipe (MA) : fl_lib/Moist Air/Elements/Pipe (MA)  length=1 m  area=pi*anode_tube_D^2/4 m^2  Dh=anode_tube_D m  length_add=0.1 m  roughness=15e-6 m  Re_lam=2000  Re_tur=4000  shape_factor=64  Nu_lam=3.66  wall_condensation=false  RH_ws=1  time_constant=1e-3 s  moisture_trace_gas_source=foundation.enum.moisture_trace_gas_source.none  moisture_source_spec=foundation.enum.moisture_source_spec.vapor  moisture_mass_flow=0 kg/s  moisture_temperature_spec=foundation.enum.temperature_spec.atmospheric  moisture_temperature=293.15 K  trace_gas_mass_flow=0 kg/s  trace_gas_temperature_spec=foundation.enum.temperature_spec.atmospheric  trace_gas_temperature=293.15 K  p_I_specify=on  p_I_priority=High  p_I=env_p MPa  p_I_nominal_specify=off  p_I_nominal_unit=MPa  p_I_nominal_value=1  T_I_specify=on  T_I_priority=High  T_I=env_T degC  T_I_nominal_specify=off  T_I_nominal_unit=K  T_I_nominal_value=1  RH_I_specify=off  RH_I_priority=High  RH_I=0  RH_I_nominal_specify=off  RH_I_nominal_unit=1  RH_I_nominal_value=1  x_w_I_specify=off  x_w_I_priority=None  x_w_I=0  x_w_I_nominal_specify=off  x_w_I_nominal_unit=1  x_w_I_nominal_value=1  y_w_I_specify=off  y_w_I_priority=None  y_w_I=0  y_w_I_nominal_specify=off  y_w_I_nominal_unit=1  y_w_I_nominal_value=1  HR_I_specify=off  HR_I_priority=None  HR_I=0  HR_I_nominal_specify=off  HR_I_nominal_unit=1  HR_I_nominal_value=1  x_g_I_specify=on  x_g_I_priority=None  x_g_I=0  x_g_I_nominal_specify=off  x_g_I_nominal_unit=1  x_g_I_nominal_value=1  y_g_I_specify=on  y_g_I_priority=High  y_g_I=tank_yH2  y_g_I_nominal_specify=off  y_g_I_nominal_unit=1  y_g_I_nominal_value=1
  Pressure Relief Valve : Subsystem  Tag=PublishSubsystem  mask(Pressure Relief Valve){D=anode_tube_D, r_min=1e-4, r_max=0.8, p_range=0.005}
      mask prompts: D "Connecting tube diameter (m)"; r_min "Min diameter ratio"; r_max "Max diameter ratio"; p_range "Pressure regulation range (MPa)"
      mask help: This subsystem models a pressure relief valve that maintains a set pressure at port A. The valve is normally closed. When the pressure is above the set pressure, it begins to open.
  Simulink-PS Converter : nesl_utility/Simulink-PS Converter  PhysicalDomain=network_engine_domain  SubClassName=ps_input  LeftPortType=input  RightPortType=output  PseudoPeriodic=off  Frequencies=[]  NoiseDistribution=none  NoiseParameters=[]  Unit=MPa  AffineConversion=off  FilteringAndDerivatives=provide  SimscapeFilterOrder=1  InputFilterTimeConstant=0.001  UdotUserProvided=0
  Simulink-PS Converter1 : nesl_utility/Simulink-PS Converter  Commented=on  PhysicalDomain=network_engine_domain  SubClassName=ps_input  LeftPortType=input  RightPortType=output  PseudoPeriodic=off  Frequencies=[]  NoiseDistribution=none  NoiseParameters=[]  Unit=1  AffineConversion=off  FilteringAndDerivatives=provide  SimscapeFilterOrder=1  InputFilterTimeConstant=0.001  UdotUserProvided=0
  Stack Pressure : Constant  Value=0.2
  Sum : Sum  Inputs=++|
  Valve : fl_lib/Moist Air/Elements/Local Restriction (MA)  Commented=on  restriction_type=foundation.enum.restriction_type.variable  restriction_area=0.001 m^2  min_area=pi*(1e-4*anode_tube_D)^2/4 m^2  max_area=pi*(0.8*anode_tube_D)^2/4 m^2  area=pi*anode_tube_D^2/4 m^2  Cd=0.64  B_lam=0.999
  A : PMIOPort  Side=Left
  wires:
  Stack Pressure/1 -> Sum/1
  Sum/1 -> Simulink-PS Converter/1
  Constant1/1 -> Sum/2
  From/1 -> Simulink-PS Converter1/1
  connections:
  Simulink-PS Converter/RConn1 -- Pressure Relief Valve/LConn2
  Environment Temperature/LConn1 -- Convective Heat Transfer/RConn1
  Convective Heat Transfer/LConn1 -- Pipe (MA)/LConn2
  A/RConn1 -- Pipe (MA)/LConn1
  Simulink-PS Converter1/RConn1 -- Valve/LConn2
  Pressure Relief Valve/LConn1 -- Pipe (MA)/RConn1
  Environment/LConn1 -- Pressure Relief Valve/RConn1

== system Fuel_Cell/Anode Gas Channels ==
  Pipe (MA) : fl_lib/Moist Air/Elements/Pipe (MA)  length=sqrt(stack_area) / 2 cm  area=stack_w_channels^2 * stack_num_channels * stack_num_cells cm^2  Dh=stack_w_channels cm  length_add=1 cm  roughness=15e-6 m  Re_lam=2000  Re_tur=4000  shape_factor=64  Nu_lam=3.66  wall_condensation=false  RH_ws=1  time_constant=1e-3 s  moisture_trace_gas_source=foundation.enum.moisture_trace_gas_source.none  moisture_source_spec=foundation.enum.moisture_source_spec.vapor  moisture_mass_flow=0 kg/s  moisture_temperature_spec=foundation.enum.temperature_spec.atmospheric  moisture_temperature=293.15 K  trace_gas_mass_flow=0 kg/s  trace_gas_temperature_spec=foundation.enum.temperature_spec.atmospheric  trace_gas_temperature=293.15 K  p_I_specify=on  p_I_priority=High  p_I=env_p MPa  p_I_nominal_specify=off  p_I_nominal_unit=MPa  p_I_nominal_value=1  T_I_specify=on  T_I_priority=High  T_I=env_T degC  T_I_nominal_specify=off  T_I_nominal_unit=K  T_I_nominal_value=1  RH_I_specify=off  RH_I_priority=High  RH_I=0  RH_I_nominal_specify=off  RH_I_nominal_unit=1  RH_I_nominal_value=1  x_w_I_specify=off  x_w_I_priority=None  x_w_I=0  x_w_I_nominal_specify=off  x_w_I_nominal_unit=1  x_w_I_nominal_value=1  y_w_I_specify=off  y_w_I_priority=None  y_w_I=0  y_w_I_nominal_specify=off  y_w_I_nominal_unit=1  y_w_I_nominal_value=1  HR_I_specify=off  HR_I_priority=None  HR_I=0  HR_I_nominal_specify=off  HR_I_nominal_unit=1  HR_I_nominal_value=1  x_g_I_specify=on  x_g_I_priority=None  x_g_I=0  x_g_I_nominal_specify=off  x_g_I_nominal_unit=1  x_g_I_nominal_value=1  y_g_I_specify=on  y_g_I_priority=High  y_g_I=tank_yH2  y_g_I_nominal_specify=off  y_g_I_nominal_unit=1  y_g_I_nominal_value=1
  Pipe (MA)1 : fl_lib/Moist Air/Elements/Pipe (MA)  length=sqrt(stack_area) / 2 cm  area=stack_w_channels^2 * stack_num_channels * stack_num_cells cm^2  Dh=stack_w_channels cm  length_add=1 cm  roughness=15e-6 m  Re_lam=2000  Re_tur=4000  shape_factor=64  Nu_lam=3.66  wall_condensation=false  RH_ws=1  time_constant=1e-3 s  moisture_trace_gas_source=foundation.enum.moisture_trace_gas_source.controlled  moisture_source_spec=foundation.enum.moisture_source_spec.vapor  moisture_mass_flow=0 kg/s  moisture_temperature_spec=foundation.enum.temperature_spec.atmospheric  moisture_temperature=293.15 K  trace_gas_mass_flow=0 kg/s  trace_gas_temperature_spec=foundation.enum.temperature_spec.atmospheric  trace_gas_temperature=293.15 K  p_I_specify=on  p_I_priority=High  p_I=env_p MPa  p_I_nominal_specify=off  p_I_nominal_unit=MPa  p_I_nominal_value=1  T_I_specify=on  T_I_priority=High  T_I=env_T degC  T_I_nominal_specify=off  T_I_nominal_unit=K  T_I_nominal_value=1  RH_I_specify=off  RH_I_priority=High  RH_I=0  RH_I_nominal_specify=off  RH_I_nominal_unit=1  RH_I_nominal_value=1  x_w_I_specify=off  x_w_I_priority=None  x_w_I=0  x_w_I_nominal_specify=off  x_w_I_nominal_unit=1  x_w_I_nominal_value=1  y_w_I_specify=off  y_w_I_priority=None  y_w_I=0  y_w_I_nominal_specify=off  y_w_I_nominal_unit=1  y_w_I_nominal_value=1  HR_I_specify=off  HR_I_priority=None  HR_I=0  HR_I_nominal_specify=off  HR_I_nominal_unit=1  HR_I_nominal_value=1  x_g_I_specify=on  x_g_I_priority=None  x_g_I=0  x_g_I_nominal_specify=off  x_g_I_nominal_unit=1  x_g_I_nominal_value=1  y_g_I_specify=on  y_g_I_priority=High  y_g_I=tank_yH2  y_g_I_nominal_specify=off  y_g_I_nominal_unit=1  y_g_I_nominal_value=1
      settings: InternalSimscapePortConfiguration="{\"Bottom\":[],\"Left\":[{\"id\":\"A\",\"label\":\"A\",\"type\":\"foundation.moist_air.moist_air\"},{\"id\":\"H\",\"label\":\"H\",\"type\":\"foundation.thermal.thermal\"},{\"id\":\"S\",\"label\":\"S\",\"type\":\"foundation.moist_air.moist_air_source\"}],\"Right\":[{\"id\":\"B\",\"label\":\"B\",\"type\":\"foundation.moist_air.moist_air\"},{\"id\":\"W\",\"label\":\"W\",\"type\":\"output\"},{\"id\":\"F\",\"label\":\"F\",\"type\":\"output\"}],\"Top\":[]}"
  in : PMIOPort  Side=Left
  out : PMIOPort  Port=2  Side=Left
  A : PMIOPort  Port=3  Side=Right
  SA : PMIOPort  Port=4  Side=Right
  FAi : PMIOPort  Port=5  Side=Right
  FAo : PMIOPort  Port=6  Side=Right
  H : PMIOPort  Port=7  Side=Right
  connections:
  A/RConn1 -- Pipe (MA)1/LConn1 -- Pipe (MA)/RConn1
  Pipe (MA)1/LConn3 -- SA/RConn1
  Pipe (MA)/RConn3 -- FAi/RConn1
  FAo/RConn1 -- Pipe (MA)1/RConn3
  H/RConn1 -- Pipe (MA)1/LConn2 -- Pipe (MA)/LConn2
  Pipe (MA)1/RConn1 -- out/RConn1
  Pipe (MA)/LConn1 -- in/RConn1

== system Fuel_Cell/Cathode Humidifier ==
  Constant Volume Chamber (MA) : fl_lib/Moist Air/Elements/Constant Volume Chamber (MA)  volume=1 l  num_ports=foundation.enum.num_ports.two  area_A=pi*anode_tube_D^2/4 m^2  area_B=pi*anode_tube_D^2/4 m^2  area_C=0.01 m^2  area_D=0.01 m^2  RH_ws=1  time_constant=1e-3 s  moisture_trace_gas_source=foundation.enum.moisture_trace_gas_source.controlled  moisture_source_spec=foundation.enum.moisture_source_spec.vapor  moisture_mass_flow=0 kg/s  moisture_temperature_spec=foundation.enum.temperature_spec.atmospheric  moisture_temperature=293.15 K  trace_gas_mass_flow=0 kg/s  trace_gas_temperature_spec=foundation.enum.temperature_spec.atmospheric  trace_gas_temperature=293.15 K  p_I_specify=on  p_I_priority=High  p_I=0.301325 MPa  p_I_nominal_specify=off  p_I_nominal_unit=MPa  p_I_nominal_value=1  T_I_specify=on  T_I_priority=High  T_I=env_T degC  T_I_nominal_specify=off  T_I_nominal_unit=K  T_I_nominal_value=1  RH_I_specify=off  RH_I_priority=High  RH_I=0  RH_I_nominal_specify=off  RH_I_nominal_unit=1  RH_I_nominal_value=1  x_w_I_specify=off  x_w_I_priority=None  x_w_I=0  x_w_I_nominal_specify=off  x_w_I_nominal_unit=1  x_w_I_nominal_value=1  y_w_I_specify=off  y_w_I_priority=None  y_w_I=0  y_w_I_nominal_specify=off  y_w_I_nominal_unit=1  y_w_I_nominal_value=1  HR_I_specify=off  HR_I_priority=None  HR_I=0  HR_I_nominal_specify=off  HR_I_nominal_unit=1  HR_I_nominal_value=1  x_g_I_specify=off  x_g_I_priority=None  x_g_I=0  x_g_I_nominal_specify=off  x_g_I_nominal_unit=1  x_g_I_nominal_value=1  y_g_I_specify=on  y_g_I_priority=High  y_g_I=tank_yH2  y_g_I_nominal_specify=off  y_g_I_nominal_unit=1  y_g_I_nominal_value=1
      settings: InternalSimscapePortConfiguration="{\"Bottom\":[],\"Left\":[{\"id\":\"A\",\"label\":\"A\",\"type\":\"foundation.moist_air.moist_air\"},{\"id\":\"B\",\"label\":\"B\",\"type\":\"foundation.moist_air.moist_air\"}],\"Right\":[{\"id\":\"W\",\"label\":\"W\",\"type\":\"output\"},{\"id\":\"F\",\"label\":\"F\",\"type\":\"output\"},{\"id\":\"H\",\"label\":\"H\",\"type\":\"foundation.thermal.thermal\"},{\"id\":\"S\",\"label\":\"S\",\"type\":\"foundation.moist_air.moist_air_source\"}],\"Top\":[]}"
  Controlled Moisture Source (MA) : fl_lib/Moist Air/Sources/Moisture & Trace Gas Sources/Moisture Source (MA)  source_type=foundation.enum.constant_controlled.controlled  moisture_source_spec=foundation.enum.moisture_source_spec.vapor  moisture_mass_flow=0 kg/s  temperature_spec=foundation.enum.temperature_spec.atmospheric  moisture_temperature=293.15 K  Phi_S_specify=off  Phi_S_priority=None  Phi_S=0 kW  Phi_S_nominal_specify=off  Phi_S_nominal_unit=kW  Phi_S_nominal_value=1  mdot_w_S_specify=off  mdot_w_S_priority=None  mdot_w_S=0 kg/s  mdot_w_S_nominal_specify=off  mdot_w_S_nominal_unit=kg/s  mdot_w_S_nominal_value=1
      settings: InternalSimscapePortConfiguration="{\"Bottom\":[],\"Left\":[{\"id\":\"S\",\"label\":\"S\",\"type\":\"foundation.moist_air.moist_air_source\"}],\"Right\":[{\"id\":\"M\",\"label\":\"M\",\"type\":\"input\"},{\"id\":\"T\",\"label\":\"T\",\"type\":\"input\"}],\"Top\":[]}"
  Convective Heat Transfer : fl_lib/Thermal/Thermal Elements/Convective Heat Transfer  thermal_type=foundation.enum.constant_variable.constant  area=0.5 m^2  heat_tr_coeff=900 W/(m^2 * K)  min_heat_tr_coeff=1e-3 W/(K*m^2)  T_specify=off  T_priority=None  T=0 K  T_nominal_specify=off  T_nominal_unit=K  T_nominal_value=1  Q_specify=off  Q_priority=None  Q=0 W  Q_nominal_specify=off  Q_nominal_unit=W  Q_nominal_value=1
  Delay One Step : Delay  DelayLength=1
  Environment Temperature : fl_lib/Thermal/Thermal Sources/Temperature Source  temperature=env_T degC
  Simulink-PS Converter : nesl_utility/Simulink-PS Converter  PhysicalDomain=network_engine_domain  SubClassName=ps_input  LeftPortType=input  RightPortType=output  PseudoPeriodic=off  Frequencies=[]  NoiseDistribution=none  NoiseParameters=[]  Unit=kg/s  AffineConversion=off  FilteringAndDerivatives=provide  SimscapeFilterOrder=1  InputFilterTimeConstant=0.001  UdotUserProvided=0
  Simulink-PS Converter1 : nesl_utility/Simulink-PS Converter  PhysicalDomain=network_engine_domain  SubClassName=ps_input  LeftPortType=input  RightPortType=output  PseudoPeriodic=off  Frequencies=[]  NoiseDistribution=none  NoiseParameters=[]  Unit=degC  AffineConversion=on  FilteringAndDerivatives=provide  SimscapeFilterOrder=1  InputFilterTimeConstant=0.001  UdotUserProvided=0
  A : PMIOPort  Side=Right
  B : PMIOPort  Port=2  Side=Left
  wires:
  Delay One Step/1 -> Simulink-PS Converter1/1
  [O2_cl_H] -> Simulink-PS Converter/1
  [T_stack] -> Delay One Step/1
  connections:
  Environment Temperature/LConn1 -- Convective Heat Transfer/RConn1
  B/RConn1 -- Constant Volume Chamber (MA)/LConn1
  A/RConn1 -- Constant Volume Chamber (MA)/LConn2
  Controlled Moisture Source (MA)/LConn1 -- Constant Volume Chamber (MA)/RConn4
  Convective Heat Transfer/LConn1 -- Constant Volume Chamber (MA)/RConn3
  Simulink-PS Converter/RConn1 -- Controlled Moisture Source (MA)/RConn1
  Controlled Moisture Source (MA)/RConn2 -- Simulink-PS Converter1/RConn1
